simulink model "Counterbalance_Valve_Circuit"  (R2022a)
settings: Solver=VariableStepAuto  StartTime=0.0  StopTime=10.0  RelTol=1e-3
libraries: fl_lib x11, sh_lib x5, nesl_utility x5
settings Model: Creator=Moham  LastModifiedBy=Moham

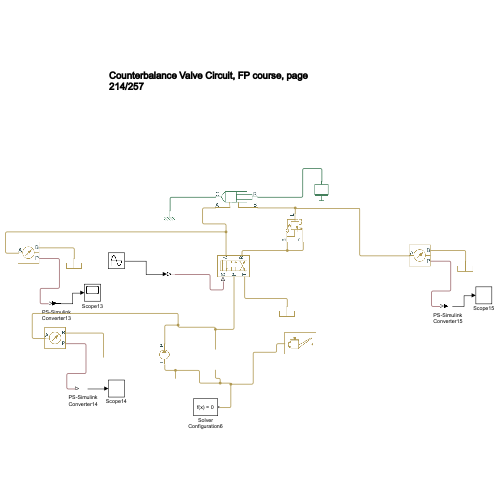
[thumbnail: Simulink's stored preview of the top-level diagram]
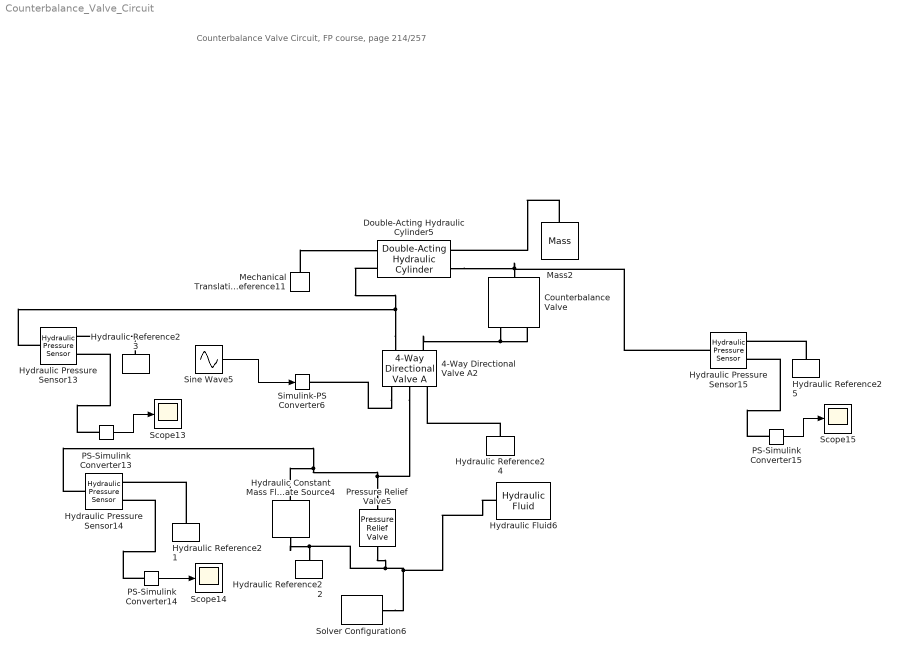
== system Counterbalance_Valve_Circuit ==
  note: Counterbalance Valve Circuit, FP course, page 214/257
  4-Way Directional Valve A2 : sh_lib/Valves/Directional Valves/4-Way Directional Valve A  mdl_type=1  area_max=0.5e-4 m^2  opening_max=0.005 m  opening_tab=[-.002, 0, .002, .005, .015] m  area_tab=[1e-09, 2.0352e-07, 4.0736e-05, .00011438, .00034356] m^2  pressure_tab=[-10000000, -5000000, -2000000, 2000000, 5000000, 10000000] Pa  flow_rate_tab=[-1e-07, -7.0711e-08, -4.4721e-08, 4.4721e-08, 7.0711e-08, 1e-07; -2.0352e-05, -1.4391e-05, -9.1017e-06, 9.1017e-06, 1.4391e-05, 2.0352e-05; -.0040736, -.0028805, -.0018218, .0018218, .0028805, .0040736; -.011438, -.0080879, -.0051152, .0051152, .0080879, .011438; -.034356, -.024293, -.015364, .015364, .024293, .034356] m^3/s  interp_method=1  extrap_method=1  C_d=0.7  A_leak=1e-12 m^2  lam_spec=1  B_lam=0.999  Re_cr=12  x_0_P_A=-2.5e-3 m  x_0_P_B=-2.5e-3 m  x_0_A_T=-2.5e-3 m  x_0_B_T=-2.5e-3 m  x_0_P_T1=2.5e-3 m  x_0_T1_T=2.5e-3 m
      settings: SourceProductBaseCode=SH  InternalSimscapePortConfiguration="{\"Bottom\":[],\"Left\":[{\"id\":\"A\",\"label\":\"A\",\"type\":\"foundation.hydraulic.hydraulic\"},{\"id\":\"B\",\"label\":\"B\",\"type\":\"foundation.hydraulic.hydraulic\"}],\"Right\":[{\"id\":\"S\",\"label\":\"S\",\"type\":\"input\"},{\"id\":\"P\",\"label\":\"P\",\"type\":\"foundation.hydraulic.hydraulic\"},{\"id\":\"T\",\"label\":\"T\",\"type\":\"foundation.hydraulic.hydraulic\"}],\"Top\":[]}"
  Counterbalance Valve : sh_lib/Valves/Flow Control Valves/Counterbalance Valve  pres_set=10e5 Pa  spring_cp=1e8 Pa/m  p_ratio=3  back_ratio=4  time_const=0.06 s  A_leak=1e-9 m^2  mdl_type=1  or_area_max=8e-5 m^2  or_opening_max=5e-3 m  opening_tab=[-.002, 0, .005, .015] m  area_tab=[1e-09, 4e-09, 1e-05, 1.02e-05] m^2  interp_method=simscape.enum.interpolation.linear  extrap_method=simscape.enum.extrapolation.linear  or_C_d=0.7  or_lam_spec=1  or_B_lam=0.999  or_Re_cr=12  check_area_max=1e-4 m^2  check_pres_crack=0.3e5 Pa  check_pres_max=1.2e5 Pa  check_C_d=0.7  check_lam_spec=1  check_B_lam=0.999  check_Re_cr=12
      settings: SourceProductBaseCode=SH  InternalSimscapePortConfiguration="{\"Bottom\":[],\"Left\":[{\"id\":\"B\",\"label\":\"B\",\"type\":\"foundation.hydraulic.hydraulic\"},{\"id\":\"P\",\"label\":\"P\",\"type\":\"foundation.hydraulic.hydraulic\"}],\"Right\":[{\"id\":\"L\",\"label\":\"L\",\"type\":\"foundation.hydraulic.hydraulic\"}],\"Top\":[]}"
  Double-Acting Hydraulic Cylinder5 : sh_lib/Hydraulic Cylinders/Double-Acting Hydraulic Cylinder  area_A=1e-3 m^2  area_B=0.5e-3 m^2  stroke=0.1 m  dead_vol_A=1e-4 m^3  dead_vol_B=1e-4 m^3  k_sh=1.4  or=sh.cylinders.enum.MechOrientationTranslational.Positive  stiff=1e6 N/m  D=150 N*s/m  hardstop_model=1  transition=0.1 mm  displacement_spec=foundation.enum.DisplacementSpec.Calculate  init_pos=0 m  init_pressure_A=0 Pa  init_pressure_B=0 Pa
      settings: SourceProductBaseCode=SH  LogSimulationData=on  InternalSimscapePortConfiguration="{\"Bottom\":[],\"Left\":[{\"id\":\"C\",\"label\":\"C\",\"type\":\"foundation.mechanical.translational.translational\"},{\"id\":\"A\",\"label\":\"A\",\"type\":\"foundation.hydraulic.hydraulic\"}],\"Right\":[{\"id\":\"R\",\"label\":\"R\",\"type\":\"foundation.mechanical.translational.translational\"},{\"id\":\"B\",\"label\":\"B\",\"type\":\"foundation.hydraulic.hydraulic\"}],\"Top\":[]}"
  Hydraulic Constant Mass Flow Rate Source4 : fl_lib/Hydraulic/Hydraulic Sources/Hydraulic Constant Mass Flow Rate Source  commanded_mass_flow=6.21 kg/s
      settings: SourceProductBaseCode=PW,SS,VE  InternalSimscapePortConfiguration="{\"Bottom\":[],\"Left\":[{\"id\":\"P\",\"label\":\"P\",\"type\":\"foundation.hydraulic.hydraulic\"}],\"Right\":[{\"id\":\"T\",\"label\":\"T\",\"type\":\"foundation.hydraulic.hydraulic\"}],\"Top\":[]}"
  Hydraulic Fluid6 : sh_lib/Hydraulic Utilities/Hydraulic Fluid  SelFluid=16  SysTemp=40  TrapAir=0.005  ViscDerFactor=1  range_error=2
  Hydraulic Pressure Sensor13 : fl_lib/Hydraulic/Hydraulic Sensors/Hydraulic Pressure Sensor
      settings: SourceProductBaseCode=PW,SS,VE
  Hydraulic Pressure Sensor14 : fl_lib/Hydraulic/Hydraulic Sensors/Hydraulic Pressure Sensor
      settings: SourceProductBaseCode=PW,SS,VE
  Hydraulic Pressure Sensor15 : fl_lib/Hydraulic/Hydraulic Sensors/Hydraulic Pressure Sensor
      settings: SourceProductBaseCode=PW,SS,VE
  Hydraulic Reference{21..25} (5 alike) : fl_lib/Hydraulic/Hydraulic Elements/Hydraulic Reference
      settings: SourceProductBaseCode=PW,SS,VE
  Mass2 : fl_lib/Mechanical/Translational Elements/Mass  mass=300 kg  num_ports=foundation.enum.numPorts2.one  v_specify=off  v_priority=High  v=0 m/s  v_nominal_specify=off  v_nominal_unit=m/s  v_nominal_value=1  f_specify=off  f_priority=None  f=0 N  f_nominal_specify=off  f_nominal_unit=N  f_nominal_value=1
      settings: SourceProductBaseCode=PW,SS,VE
  Mechanical Translational Reference11 : fl_lib/Mechanical/Translational Elements/Mechanical Translational Reference
      settings: SourceProductBaseCode=PW,SS,VE
  PS-Simulink Converter13 : nesl_utility/PS-Simulink Converter  PhysicalDomain=network_engine_domain  SubClassName=ps_output  LeftPortType=input  RightPortType=output  PseudoPeriodic=off  Frequencies=[]  VectorFormat=inherit  Unit=inherit  AffineConversion=off
      settings: SourceProductBaseCode=SS,PW,VE
  PS-Simulink Converter14 : nesl_utility/PS-Simulink Converter  PhysicalDomain=network_engine_domain  SubClassName=ps_output  LeftPortType=input  RightPortType=output  PseudoPeriodic=off  Frequencies=[]  VectorFormat=inherit  Unit=inherit  AffineConversion=off
      settings: SourceProductBaseCode=SS,PW,VE
  PS-Simulink Converter15 : nesl_utility/PS-Simulink Converter  PhysicalDomain=network_engine_domain  SubClassName=ps_output  LeftPortType=input  RightPortType=output  PseudoPeriodic=off  Frequencies=[]  VectorFormat=inherit  Unit=inherit  AffineConversion=off
      settings: SourceProductBaseCode=SS,PW,VE
  Pressure Relief Valve5 : sh_lib/Valves/Pressure Control Valves/Pressure Relief Valve  valve_area_spec=1  p_diff_TLU=[30.15e5 : 15e3 : 31.35e5] Pa  area_TLU=[1 : 1 : 9] .* 1e-5 m^2  area_max=1e-4 m^2  pres_set=50e5 Pa  reg_range=5e5 Pa  C_d=0.7  A_leak=1e-12 m^2  lam_spec=1  B_lam=0.999  Re_cr=12  dynamic=0  tau=0.1 s  area_init=1e-12 m^2
      settings: SourceProductBaseCode=SH  InternalSimscapePortConfiguration="{\"Bottom\":[],\"Left\":[{\"id\":\"A\",\"label\":\"A\",\"type\":\"foundation.hydraulic.hydraulic\"}],\"Right\":[{\"id\":\"B\",\"label\":\"B\",\"type\":\"foundation.hydraulic.hydraulic\"}],\"Top\":[]}"
  Scope13 : Scope
  Scope14 : Scope
  Scope15 : Scope
  Simulink-PS Converter6 : nesl_utility/Simulink-PS Converter  PhysicalDomain=network_engine_domain  SubClassName=ps_input  LeftPortType=input  RightPortType=output  PseudoPeriodic=off  Frequencies=[]  NoiseDistribution=none  NoiseParameters=[]  Unit=1  AffineConversion=off  FilteringAndDerivatives=provide  SimscapeFilterOrder=1  InputFilterTimeConstant=0.001  UdotUserProvided=0
      settings: SourceProductBaseCode=SS,PW,VE
  Sine Wave5 : Sin  Amplitude=0.003  SampleTime=0
  Solver Configuration6 : nesl_utility/Solver Configuration  PhysicalDomain=network_engine_domain  SubClassName=solver  LeftPortType=input  RightPortType=generic  Tones=[]  Harmonics=[]  SimulateNoise=off  Profile=off  UseLocalSampling=off  EnableSwitchedLinearOptims=on  FrequencyDomain=off  UseCCode=off  RelTol=0.001  AbsTol=1e-06  MinStep=1e-09  ToWorkspace=off  RevertToSquareIcSolve=off  NumHomotopyIterations=100  PhasorMode=off  PhasorModeNumHarmonics=1  IndexReductionMethod=DerivativeReplacement  DoDC=off  ResidualTolerance=1e-09  UseLocalSolver=off  LocalSolverChoice=NE_BACKWARD_EULER_ADVANCER  LocalSolverSampleTime=0.001  DoFixedCost=off  MaxNonlinIter=3  MaxModeIter=2  ComputeImpulses=off  ImpulseIterations=2  LinearAlgebra=auto  LinearAlgebraNumThread=0  EquationFormulation=NE_TIME_EF  DelaysMemoryBudget=1024  AutomaticFiltering=on  FilteringTimeConstant=0.001  PartitionStorageMethod=AS_NEEDED  PartitionMemoryBudget=1024  PartitionMethod=ROBUST
      settings: SourceProductBaseCode=SS,PW,VE
  wires:
  PS-Simulink Converter13/1 -> Scope13/1
  PS-Simulink Converter14/1 -> Scope14/1
  PS-Simulink Converter15/1 -> Scope15/1
  Sine Wave5/1 -> Simulink-PS Converter6/1
  connections:
  Counterbalance Valve/RConn1 -- Double-Acting Hydraulic Cylinder5/RConn2 -- Hydraulic Pressure Sensor15/LConn1
  Hydraulic Constant Mass Flow Rate Source4/RConn1 -- Hydraulic Reference22/LConn1 -- Pressure Relief Valve5/RConn1 -- Hydraulic Fluid6/RConn1 -- Solver Configuration6/RConn1
  Hydraulic Pressure Sensor14/LConn1 -- Hydraulic Constant Mass Flow Rate Source4/LConn1 -- 4-Way Directional Valve A2/RConn2 -- Pressure Relief Valve5/LConn1
  4-Way Directional Valve A2/LConn1 -- Double-Acting Hydraulic Cylinder5/LConn2 -- Hydraulic Pressure Sensor13/LConn1
  Counterbalance Valve/LConn1 -- 4-Way Directional Valve A2/LConn2 -- Counterbalance Valve/LConn2
  Mass2/LConn1 -- Double-Acting Hydraulic Cylinder5/RConn1
  PS-Simulink Converter15/LConn1 -- Hydraulic Pressure Sensor15/RConn2
  Hydraulic Reference25/LConn1 -- Hydraulic Pressure Sensor15/RConn1
  PS-Simulink Converter14/LConn1 -- Hydraulic Pressure Sensor14/RConn2
  Hydraulic Reference24/LConn1 -- 4-Way Directional Valve A2/RConn3
  Hydraulic Reference23/LConn1 -- Hydraulic Pressure Sensor13/RConn1
  PS-Simulink Converter13/LConn1 -- Hydraulic Pressure Sensor13/RConn2
  Hydraulic Reference21/LConn1 -- Hydraulic Pressure Sensor14/RConn1
  4-Way Directional Valve A2/RConn1 -- Simulink-PS Converter6/RConn1
  Mechanical Translational Reference11/LConn1 -- Double-Acting Hydraulic Cylinder5/LConn1
